simulink model "Vehicle_Model"  (R2025b)
settings: Solver=VariableStepAuto  StartTime=0.0  StopTime=10.0  RelTol=1e-3
undefined symbols (not defined in the file): tirPath
settings Model: Creator=alphabet1671  LastModifiedBy=alphabet1671

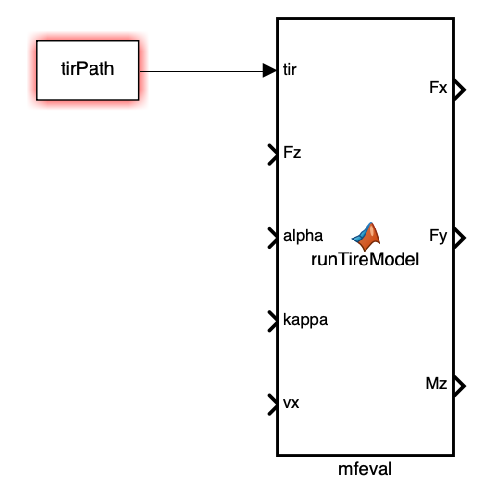
[thumbnail: Simulink's stored preview of the top-level diagram]
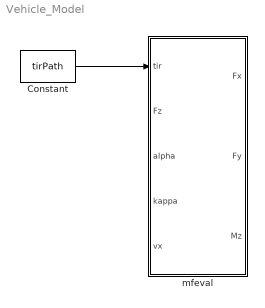
== system Vehicle_Model ==
  Constant : Constant  Value=tirPath  VectorParams1D=off
  mfeval : MATLAB Function  TreatAsAtomicUnit=on
  wires:
  Constant/1 -> mfeval/1(tir)

== matlab function Vehicle_Model/mfeval ==
  data: Fx output; Fy output; tir input; Fz input; alpha input; kappa input; vx input; Mz output
function [Fx, Fy, Mz]= runTireModel(tir, Fz, alpha, kappa, vx)

tire = readTIR(tir);

inputs = [Fz, kappa, alpha, 0, 0, vx];

outputs = mfeval(inputs, tire, 121);

Fx = outputs.Fx;
Fy = outputs.Fy;
Mz = outputs.Mz;

end
